simulink model "Model"  (R2023b)
settings: Solver=VariableStepAuto  StartTime=0.0  StopTime=1  RelTol=1e-3
values from neighbouring files (symbols this model uses):
  B = 0.0129    [PARAMETERS_MODEL_GR2.m]    (also in Parameters.m; Parameters_Chloe.m)
  J = 0.2799    [PARAMETERS_MODEL_GR2.m]    (also in Parameters.m; Parameters_Chloe.m)
  L_lr = 1.8e-3    (= 0.0018)    [PARAMETERS_MODEL_GR2.m]    (also in Parameters.m; Parameters_Chloe.m)
  L_ls = 1.8e-3    (= 0.0018)    [PARAMETERS_MODEL_GR2.m]    (also in Parameters.m; Parameters_Chloe.m)
  P = 4    [PARAMETERS_MODEL_GR2.m]    (also in Parameters.m; Parameters_Chloe.m)
  R_r = 0.1091    [PARAMETERS_MODEL_GR2.m]    (also in Parameters.m; Parameters_Chloe.m)
  R_s = 0.0629    [PARAMETERS_MODEL_GR2.m]    (also in Parameters.m; Parameters_Chloe.m)
libraries: spsSeriesRLCBranchLib x8, spsDiodeLib x6, spsIGBTDiodeLib x6, spsVoltageMeasurementLib x4, spsACVoltageSourceLib x3, spsAsynchronousMachinepuUnitsLib x1, spsTriangleGeneratorLib x1, sps_lib x1
settings Model: Creator=dimit  LastModifiedBy=dimit

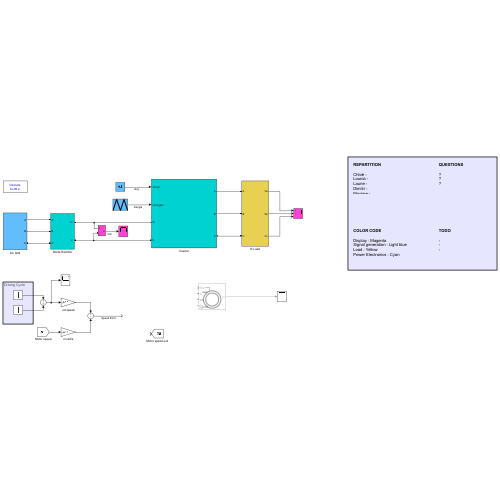
[thumbnail: Simulink's stored preview of the top-level diagram]
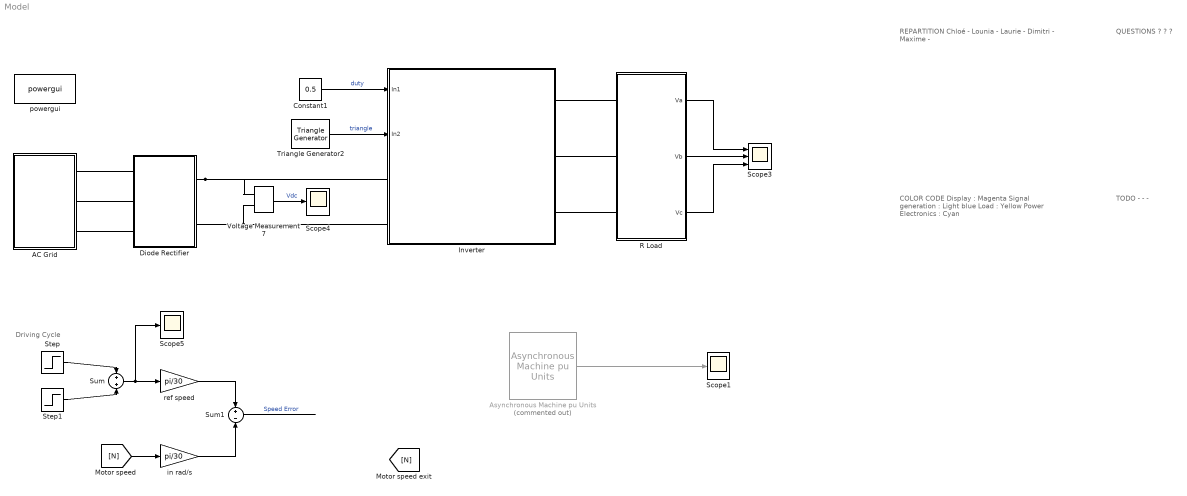
== system Model ==
  note: COLOR CODE
      |
      | Display : Magenta
      | Signal generation : Light blue
      | Load : Yellow
      | Power Electronics : Cyan
  note: Driving Cycle
  note: QUESTIONS
      |
      | ?
      | ?
      | ?
  note: TODO
      |
      | -
      | -
      | -
  note: REPARTITION
      |
      | Chloé -
      | Lounia -
      | Laurie -
      | Dimitri -
      | Maxime -
  AC Grid : Subsystem
  Asynchronous Machine pu Units : spsAsynchronousMachinepuUnitsLib/Asynchronous Machine pu Units  Commented=on  RotorType=Squirrel-cage  PresetModel=No  MechanicalLoad=Torque Tm  ShowDetailedParameters=on  ReferenceFrame=Rotor  Units=pu  MeasurementBus=on  NominalParameters=[3730 460 60]  VoltageRatio=1  Stator=[R_s L_ls]  Rotor=[R_r L_lr]  Cage1=[0.01909 0.0397]  Cage2=[0.01909 0.0397]  Lm=L_m  Mechanical=[J B P]  PolePairs=2  InitialConditions="[ 1,0   0,0,0   0,0,0 ]"  SimulateSaturation=off  Saturation="[0.212,0.4201,0.8125,1.0979,1.4799,2.2457,3.2586,4.5763,6.4763 ;   0.5,0.7,0.9,1,1.1,1.2 ,1.3,1.4,1.5]"  LoadFlowParameters=0  TsPowergui=0  TsBlock=-1  IterativeModel=Trapezoidal non iterative  IterativeDiscreteModel=Trapezoidal non iterative  Pmec=0
      settings: LibrarySourceBlock=|
      | sps_lib/Electrical Machines/Asynchronous Machine
      | pu Units
  Constant1 : Constant  Value=0.5
  Diode Rectifier : Subsystem
  Inverter : Subsystem
  R Load : Subsystem
  Scope1 : Scope
  Scope3 : Scope  NumInputPorts=3
  Scope4 : Scope
  Scope5 : Scope
  Step : Step  Time=0.1  After=1200  SampleTime=0
  Step1 : Step  Time=1.7  After=-1200  SampleTime=0
  Sum : Sum  Inputs=+|+
  Sum1 : Sum  Inputs=+|-
  Triangle Generator2 : spsTriangleGeneratorLib/Triangle Generator  Freq=10e3  Phase=0  Ts=0
  Voltage Measurement7 : spsVoltageMeasurementLib/Voltage Measurement  PhasorSimulation=off  OutputType=Complex  PSBequivalent=0
  in rad/s : Gain  Gain=pi/30
  powergui : sps_lib/powergui  Priority=1  SimulationMode=Discrete  SampleTime=1e-6  frequency=60  Iterations=50  frequencyindice=50  Pbase=100e6  ErrMax=1e-4  UnitsV=kV  UnitsW=MW  buscounter=0  FunctionMessages=off  echomessages=off  EnableUseOfTLC=off  CurrentSourceSwitches=off  DisableSnubberDevices=off  DisableRonSwitches=off  DisableVfSwitches=off  DisplayEquations=off  AutomaticDiscreteSolvers=off  SolverType=Tustin/Backward Euler (TBE)  Interpol=off  ExternalGateDelay=off  methode=off  Ts=100  x0status=blocks  SPID=on  SwTol=0  HookPort=off  NonlinearTolerance=1e-4  nMaxIteration=100  ContinueOnMaxIteration=off  RestoreLinks=warning  ResistiveCurrentMeasurement=off  Frange=[0:2:500]  Ylog=off  Xlog=on  ShowGrid=off  save=off  variable=ZData  structure=0  ZoomFFT=off  StartTime=0.0  cycles=1  DisplayStyle=1  fundamental=60  FreqAxis=off  MaxFrequency=1000  frequencyindicesteady=1  RmsSteady=1  display=off
  ref speed : Gain  Gain=pi/30
  wires:
  Triangle Generator2/1 -> Inverter/2(In2)  "triangle"
  Voltage Measurement7/1 -> Scope4/1  "Vdc"
  Constant1/1 -> Inverter/1(In1)  "duty"
  Sum1/1 -> ?  "Speed Error"
  [N] -> in rad/s/1
  Step1/1 -> Sum/2
  Sum/1 -> ref speed/1, Scope5/1
  ref speed/1 -> Sum1/1
  in rad/s/1 -> Sum1/2
  Step/1 -> Sum/1
  Asynchronous Machine pu Units/1 -> Scope1/1
  R Load/1(Va) -> Scope3/1
  R Load/2(Vb) -> Scope3/2
  R Load/3(Vc) -> Scope3/3
  connections:
  Voltage Measurement7/LConn2 -- Inverter/LConn2 -- Diode Rectifier/RConn2
  Diode Rectifier/RConn1 -- Voltage Measurement7/LConn1 -- Inverter/LConn1
  AC Grid/LConn1 -- Diode Rectifier/LConn1
  AC Grid/LConn2 -- Diode Rectifier/LConn2
  AC Grid/LConn3 -- Diode Rectifier/LConn3
  Inverter/RConn1 -- R Load/LConn1
  Inverter/RConn2 -- R Load/LConn2
  Inverter/RConn3 -- R Load/LConn3

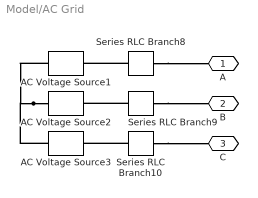
== system Model/AC Grid ==
  AC Voltage Source1 : spsACVoltageSourceLib/AC Voltage Source  Amplitude=380  Phase=0  Frequency=50  SampleTime=0  Measurements=Voltage  BusType=swing  Pref=10e3  Qref=0  Qmin=-inf  Qmax=+inf
  AC Voltage Source2 : spsACVoltageSourceLib/AC Voltage Source  Amplitude=380  Phase=120  Frequency=50  SampleTime=0  Measurements=Voltage  BusType=swing  Pref=10e3  Qref=0  Qmin=-inf  Qmax=+inf
  AC Voltage Source3 : spsACVoltageSourceLib/AC Voltage Source  Amplitude=380  Phase=240  Frequency=50  SampleTime=0  Measurements=Voltage  BusType=swing  Pref=10e3  Qref=0  Qmin=-inf  Qmax=+inf
  Series RLC Branch10 : spsSeriesRLCBranchLib/Series RLC Branch  LConnTagsString=__new0  RConnTagsString=__new0  BranchType=L  Resistance=1  Inductance=1e-3  SetiL0=off  InitialCurrent=0  Capacitance=15e-6  Setx0=off  InitialVoltage=0  Measurements=None
  Series RLC Branch8 : spsSeriesRLCBranchLib/Series RLC Branch  LConnTagsString=__new0  RConnTagsString=__new0  BranchType=L  Resistance=1  Inductance=1e-3  SetiL0=off  InitialCurrent=0  Capacitance=15e-6  Setx0=off  InitialVoltage=0  Measurements=None
  Series RLC Branch9 : spsSeriesRLCBranchLib/Series RLC Branch  LConnTagsString=__new0  RConnTagsString=__new0  BranchType=L  Resistance=1  Inductance=1e-3  SetiL0=off  InitialCurrent=0  Capacitance=15e-6  Setx0=off  InitialVoltage=0  Measurements=None
  A : PMIOPort  Side=Left
  B : PMIOPort  Port=2  Side=Left
  C : PMIOPort  Port=3  Side=Left
  connections:
  Series RLC Branch10/LConn1 -- C/RConn1
  AC Voltage Source2/LConn1 -- AC Voltage Source1/LConn1 -- AC Voltage Source3/LConn1
  Series RLC Branch8/LConn1 -- A/RConn1
  Series RLC Branch8/RConn1 -- AC Voltage Source1/RConn1
  Series RLC Branch9/RConn1 -- AC Voltage Source2/RConn1
  Series RLC Branch10/RConn1 -- AC Voltage Source3/RConn1
  Series RLC Branch9/LConn1 -- B/RConn1

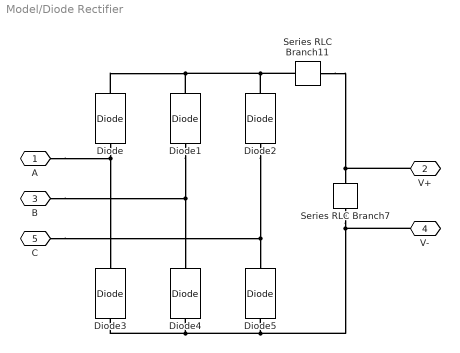
== system Model/Diode Rectifier ==
  Diode{,1..5} (6 alike) : spsDiodeLib/Diode  Ron=0.001  Lon=0  Vf=0  IC=0  UseSnubber=0  Rs=500  Cs=250e-9  Measurements=off
  Series RLC Branch11 : spsSeriesRLCBranchLib/Series RLC Branch  LConnTagsString=__new0  RConnTagsString=__new0  BranchType=L  Resistance=1  Inductance=10e-3  SetiL0=off  InitialCurrent=0  Capacitance=15e-6  Setx0=off  InitialVoltage=0  Measurements=None
  Series RLC Branch7 : spsSeriesRLCBranchLib/Series RLC Branch  LConnTagsString=__new0  RConnTagsString=__new0  BranchType=C  Resistance=1  Inductance=1e-3  SetiL0=off  InitialCurrent=0  Capacitance=15e-3  Setx0=off  InitialVoltage=0  Measurements=None
  A : PMIOPort  Side=Left
  V+ : PMIOPort  Port=2  Side=Right
  B : PMIOPort  Port=3  Side=Left
  V- : PMIOPort  Port=4  Side=Right
  C : PMIOPort  Port=5  Side=Left
  connections:
  Diode1/LConn1 -- B/RConn1 -- Diode4/RConn1
  Series RLC Branch7/RConn1 -- V-/RConn1 -- Diode3/LConn1 -- Diode4/LConn1 -- Diode5/LConn1
  Diode2/LConn1 -- C/RConn1 -- Diode5/RConn1
  Diode/LConn1 -- A/RConn1 -- Diode3/RConn1
  Diode/RConn1 -- Series RLC Branch11/RConn1 -- Diode2/RConn1 -- Diode1/RConn1
  Series RLC Branch11/LConn1 -- V+/RConn1 -- Series RLC Branch7/LConn1

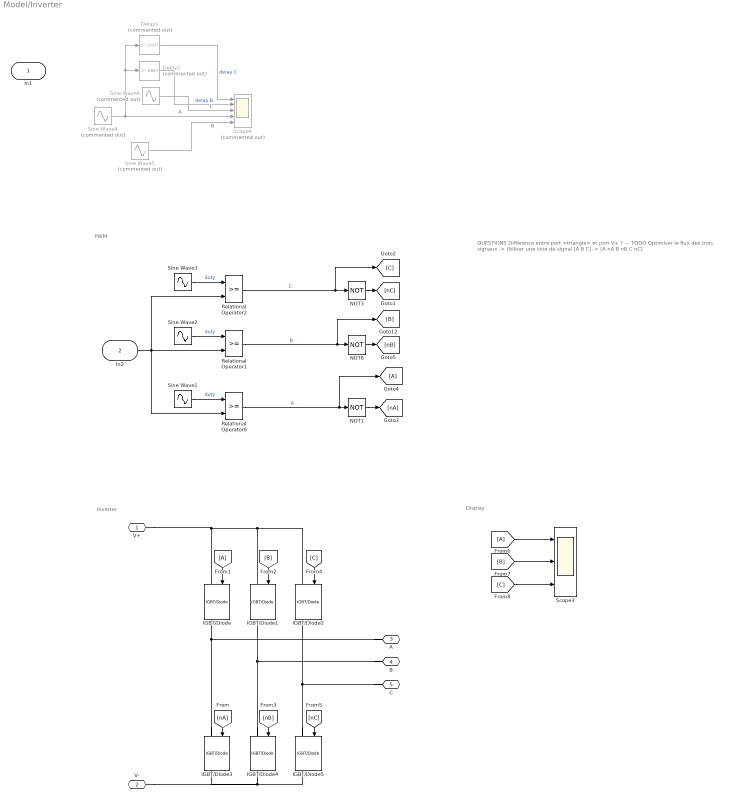
== system Model/Inverter ==
  note: Display
  note: PWM
  note: QUESTIONS
      |
      | Différence entre port <triangle> et port V+ ?
      |
      | ---
      |
      | TODO
      |
      | Optimiser le flux des trois signaux -> Utiliser une liste de signal [A B C] -> [A nA B nB C nC]
  note: Inverter
  In1 : Inport
  In2 : Inport  Port=2
  Delay1 : Delay  Commented=on  DelayLength=13333
  Delay2 : Delay  Commented=on  DelayLength=6667
  From1 : From
  From6 : From
  Goto4 : Goto
  IGBT/Diode{,1..5} (6 alike) : spsIGBTDiodeLib/IGBT//Diode  Ron=1e-3  Rs=1e5  Cs=inf  Measurements=on
  NOT1 : Logic  Operator=NOT  AllPortsSameDT=off  OutDataTypeStr=boolean
  NOT3 : Logic  Operator=NOT  AllPortsSameDT=off  OutDataTypeStr=boolean
  NOT6 : Logic  Operator=NOT  AllPortsSameDT=off  OutDataTypeStr=boolean
  Relational Operator1 : RelationalOperator  OutDataTypeStr=boolean  RndMeth=Simplest  InputSameDT=off
  Relational Operator2 : RelationalOperator  OutDataTypeStr=boolean  RndMeth=Simplest  InputSameDT=off
  Relational Operator6 : RelationalOperator  OutDataTypeStr=boolean  RndMeth=Simplest  InputSameDT=off
  Scope3 : Scope  NumInputPorts=3
  Scope4 : Scope  Commented=on  NumInputPorts=5
  Sine Wave1 : Sin  Frequency=2*pi*50  SampleTime=0
  Sine Wave2 : Sin  Frequency=2*pi*50  Phase=4*pi/3  SampleTime=0
  Sine Wave3 : Sin  Frequency=2*pi*50  Phase=2*pi/3  SampleTime=0
  Sine Wave4 : Sin  Commented=on  Frequency=2*pi*50  SampleTime=0
  Sine Wave5 : Sin  Commented=on  Frequency=2*pi*50  Phase=4*pi/3  SampleTime=0
  Sine Wave6 : Sin  Commented=on  Frequency=2*pi*50  Phase=2*pi/3  SampleTime=0
  V+ : PMIOPort  Side=Left
  V- : PMIOPort  Port=2  Side=Left
  A : PMIOPort  Port=3  Side=Right
  B : PMIOPort  Port=4  Side=Right
  C : PMIOPort  Port=5  Side=Right
  wires:
  [nA] -> IGBT/Diode3/1
  [B] -> IGBT/Diode1/1
  [C] -> IGBT/Diode2/1
  [nB] -> IGBT/Diode4/1
  From1/1 -> IGBT/Diode/1
  [nC] -> IGBT/Diode5/1
  Sine Wave3/1 -> Relational Operator2/1  "duty"
  Relational Operator1/1 -> [B], NOT6/1  "B"
  Relational Operator6/1 -> Goto4/1, NOT1/1  "A"
  Sine Wave2/1 -> Relational Operator1/1  "duty"
  Sine Wave1/1 -> Relational Operator6/1  "duty"
  Relational Operator2/1 -> [C], NOT3/1  "C"
  NOT1/1 -> [nA]
  NOT6/1 -> [nB]
  NOT3/1 -> [nC]
  Sine Wave4/1 -> Delay2/1, Delay1/1, Scope4/4  "A"
  Sine Wave5/1 -> Scope4/5  "B"
  Sine Wave6/1 -> Scope4/3  "C"
  Delay2/1 -> Scope4/2  "delay B"
  Delay1/1 -> Scope4/1  "delay C"
  In2/1 -> Relational Operator2/2, Relational Operator6/2, Relational Operator1/2
  From6/1 -> Scope3/1
  [B] -> Scope3/2
  [C] -> Scope3/3
  connections:
  IGBT/Diode5/LConn1 -- IGBT/Diode2/RConn1 -- C/RConn1
  IGBT/Diode1/LConn1 -- IGBT/Diode/LConn1 -- V+/RConn1 -- IGBT/Diode2/LConn1
  IGBT/Diode4/RConn1 -- IGBT/Diode3/RConn1 -- V-/RConn1 -- IGBT/Diode5/RConn1
  IGBT/Diode4/LConn1 -- IGBT/Diode1/RConn1 -- B/RConn1
  IGBT/Diode3/LConn1 -- IGBT/Diode/RConn1 -- A/RConn1

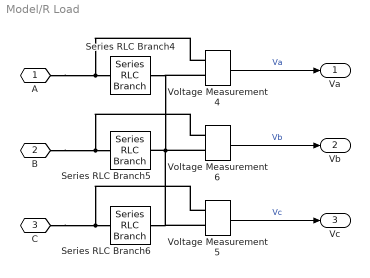
== system Model/R Load ==
  Series RLC Branch4 : spsSeriesRLCBranchLib/Series RLC Branch  LConnTagsString=__new0  RConnTagsString=__new0  BranchType=R  Resistance=1  Inductance=0  SetiL0=off  InitialCurrent=0  Capacitance=0  Setx0=off  InitialVoltage=0  Measurements=None
  Series RLC Branch5 : spsSeriesRLCBranchLib/Series RLC Branch  LConnTagsString=__new0  RConnTagsString=__new0  BranchType=R  Resistance=1  Inductance=0  SetiL0=off  InitialCurrent=0  Capacitance=0  Setx0=off  InitialVoltage=0  Measurements=None
  Series RLC Branch6 : spsSeriesRLCBranchLib/Series RLC Branch  LConnTagsString=__new0  RConnTagsString=__new0  BranchType=R  Resistance=1  Inductance=0  SetiL0=off  InitialCurrent=0  Capacitance=0  Setx0=off  InitialVoltage=0  Measurements=None
  Voltage Measurement4 : spsVoltageMeasurementLib/Voltage Measurement  PhasorSimulation=off  OutputType=Complex  PSBequivalent=0
  Voltage Measurement5 : spsVoltageMeasurementLib/Voltage Measurement  PhasorSimulation=off  OutputType=Complex  PSBequivalent=0
  Voltage Measurement6 : spsVoltageMeasurementLib/Voltage Measurement  PhasorSimulation=off  OutputType=Complex  PSBequivalent=0
  A : PMIOPort  Side=Left
  B : PMIOPort  Port=2  Side=Left
  C : PMIOPort  Port=3  Side=Left
  Va : Outport
  Vb : Outport  Port=2
  Vc : Outport  Port=3
  wires:
  Voltage Measurement5/1 -> Vc/1  "Vc"
  Voltage Measurement4/1 -> Va/1  "Va"
  Voltage Measurement6/1 -> Vb/1  "Vb"
  connections:
  Series RLC Branch5/LConn1 -- Voltage Measurement4/LConn2 -- Series RLC Branch4/LConn1 -- Voltage Measurement6/LConn2 -- Series RLC Branch6/LConn1 -- Voltage Measurement5/LConn2
  Series RLC Branch4/RConn1 -- A/RConn1 -- Voltage Measurement4/LConn1
  Series RLC Branch6/RConn1 -- C/RConn1 -- Voltage Measurement5/LConn1
  Series RLC Branch5/RConn1 -- B/RConn1 -- Voltage Measurement6/LConn1
